simulink model "Vehicle_Model_Controller_may25"  (R2020b)
settings: Solver=VariableStepAuto  StartTime=0.0  StopTime=20  FixedStep=0.015  MaxStep=0.1  RelTol=1e-3
model workspace (MAT data in the model file):
  Kp = 10
  understeer_gradient = 0.05
undefined symbols (not defined in the file or in its folder): inch2mm, S1, S2, S3, S4, steer_slope
libraries: fl_lib x24, nesl_utility x22, sdl_lib x6, autolibshared x1, autolibdatasheetbattery x1, dspstat3 x1, pid_lib x1
(part 2 of 2)

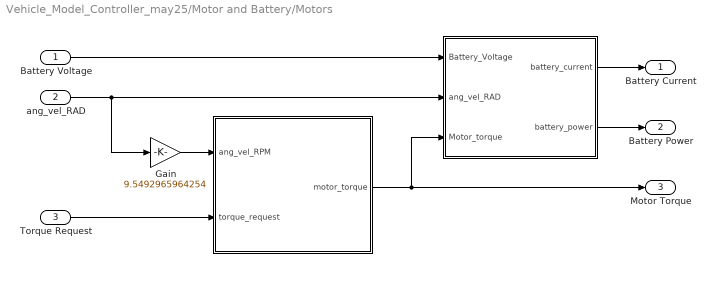
== system Vehicle_Model_Controller_may25/Motor and Battery/Motors ==
  Battery Voltage : Inport
  ang_vel_RAD : Inport  Port=2
  Torque Request : Inport  Port=3
  " " : MATLAB Function  TreatAsAtomicUnit=on
  "  " : MATLAB Function  TreatAsAtomicUnit=on
  Gain : Gain  Gain=9.5492965964254
  Battery Current : Outport
  Battery Power : Outport  Port=2
  Motor Torque : Outport  Port=3
  wires:
  Torque Request/1 -> " "/2(torque_request)
  Battery Voltage/1 -> "  "/1(Battery_Voltage)
  ang_vel_RAD/1 -> Gain/1, "  "/2(ang_vel_RAD)
  "  "/1(battery_current) -> Battery Current/1
  " "/1(motor_torque) -> Motor Torque/1, "  "/3(Motor_torque)
  "  "/2(battery_power) -> Battery Power/1
  Gain/1 -> " "/1(ang_vel_RPM)

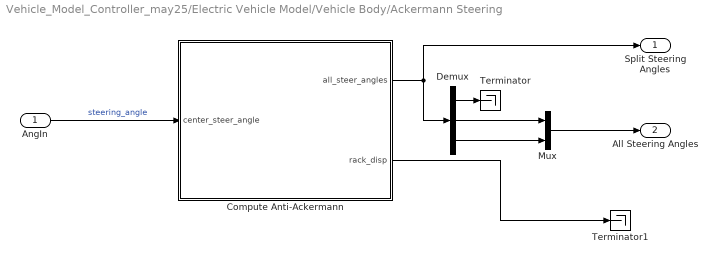
== system Vehicle_Model_Controller_may25/Electric Vehicle Model/Vehicle Body/Ackermann Steering ==
  AngIn : Inport
  Compute Anti-Ackermann : MATLAB Function  TreatAsAtomicUnit=on
  Demux : Demux  Outputs=3
  Mux : Mux  Inputs=2
  Terminator : Terminator
  Terminator1 : Terminator
  Split Steering Angles : Outport
  All Steering Angles : Outport  Port=2
  wires:
  Demux/1 -> Terminator/1
  Compute Anti-Ackermann/1(all_steer_angles) -> Demux/1, Split Steering Angles/1
  Demux/3 -> Mux/2
  AngIn/1 -> Compute Anti-Ackermann/1(center_steer_angle)  "steering_angle"
  Demux/2 -> Mux/1
  Mux/1 -> All Steering Angles/1
  Compute Anti-Ackermann/2(rack_disp) -> Terminator1/1

== matlab function Vehicle_Model_Controller_may25/Subsystem/MATLAB Function4 ==
  data: steering_angle input; torque_output output; torque_input_1 input size=[1 2]; torque_input_2 input size=[1 2]
function torque_output = cornering_torque_switcher(steering_angle, torque_input_1, torque_input_2)

if steering_angle ~= 0
    torque_output = torque_input_1;
else
    torque_output = torque_input_2;


end

== matlab function Vehicle_Model_Controller_may25/Subsystem/MATLAB Function3 ==
  data: vehicle_x_speed input; v output; vehicle_y_speed input
function v = fcn(vehicle_x_speed, vehicle_y_speed)

v = sqrt(vehicle_x_speed^2 + vehicle_y_speed^2);

== matlab function Vehicle_Model_Controller_may25/Electric Vehicle Model/Vehicle Body/Ackermann Steering/Compute Anti-Ackermann ==
  data: center_steer_angle input; all_steer_angles output size=[1 3]; S1 parameter; S2 parameter; S3 parameter; S4 parameter; inch2mm parameter; steer_slope parameter; deg2rad parameter; rack_disp output
function [all_steer_angles, rack_disp]  = anti_ackermann(center_steer_angle, S1, S2, S3, S4, inch2mm, steer_slope, deg2rad)
rack_disp = steer_slope * inch2mm * center_steer_angle;

left_steer_angle = -((S1*(-center_steer_angle)^3)+(S2*(-center_steer_angle)^2)+(S3*-center_steer_angle)+S4);
right_steer_angle = ((S1*(center_steer_angle)^3)+(S2*(center_steer_angle)^2)+(S3*center_steer_angle)+S4);

all_steer_angles = [center_steer_angle left_steer_angle right_steer_angle].*deg2rad;

end

== matlab function Vehicle_Model_Controller_may25/Motor and Battery/Motors/  ==
  data: ang_vel_RPM input; motor_torque output size=[1 2]; torque_request input
function motor_torque = get_torque(ang_vel_RPM, torque_request)
%% Actual Torque Output
% Developers:    Demetrius Gulewicz

% Developed for: Purdue Electric Racing
% Date:          09/18/2021
%
% Definitions:
% ang_vel:   Angular velocity of each wheel on the wheel fixed y axis [RPM]
% torque_request: Requested torque from the LP model                  [Nm]

%% Constants
% quadratic constants that connect current and max RPM of motors
a_v = 0.2667;
b_v = -66.353;
c_v = 10452 - ang_vel_RPM;

% quadratic constants that connnect current and max torque of motors
a_t = -0.0987;
b_t = 45.799;
c_t = -129.65;

% maximum possible current at the current RPM
max_current = [0, 0];


%% Calculate Maximum Torque Possible
% calculate the maximum current possible at the current RPM
for i = [1:2]
   if ang_vel_RPM(i) < 7000
       max_current(i) = 70;
   else
       max_current(i) = (-b_v - sqrt(b_v^2 - (4*a_v.*c_v(i)))) .* (1/(2*a_v));
   end
end

% calculate the meximum torque at the max current
max_torque = (a_t .* (max_current.^2)) + (b_t .* max_current) + c_t;
for i = [1:2]
   if max_torque(i) < 0
      max_torque(i) = 0;
   end
end

motor_torque_matrix = [max_torque; torque_request'];
motor_torque = min(motor_torque_matrix);

== matlab function Vehicle_Model_Controller_may25/Electric Vehicle Model/Vehicle Body/MATLAB Function ==
  data: Vy input; Vx input; Fext output
function Fext = get_downforce(Vy, Vx)
%% Constants
rho = 1.225; % Air density [Kg/m^3]
cl = 2.11014; % Lift coefficient [unitless]
A = 1.0221; % Frontal Area [m^2]


%% Computation
% Compute CoG Velocity
Vcog = Vx^2 + Vy^2;

% Compute DownForce
Fz = 0.5 * rho * Vcog * cl * A;
Fext = [0, 0, Fz];

== matlab function Vehicle_Model_Controller_may25/Electric Vehicle Model/MATLAB Function ==
  data: FwF output; FX input; FwR output
function [FwF, FwR] = fcn(FX)
%% Construct Force Matrix
FwF = FX(1:2);
FwR = FX(3:4);

== matlab function Vehicle_Model_Controller_may25/Subsystem/MATLAB Function ==
  data: driver_steering_angle output; vehicle_speed input; driver_steering_angle input; desired_wheelspeed output double
function [driver_steering_angle, desired_wheelspeed]  = wheel_speed_calculation(vehicle_speed, driver_steering_angle)
% desired_wheelspeed: 1 * 2 array [rl, rr]
% driver_steering_angle: 1 * angle variable
% vehicle_speed: 1 * VB CoG X-Velocity variable

W = 1.269; % m
L = 1.574; % m

ground_speed_rl = vehicle_speed + vehicle_speed * W * tan(driver_steering_angle) / (2*L);
ground_speed_rr = vehicle_speed - vehicle_speed * W * tan(driver_steering_angle) / (2*L);
desired_wheelspeed = [ground_speed_rl, ground_speed_rr];

== matlab function Vehicle_Model_Controller_may25/Subsystem/MATLAB Function1 ==
  data: measured_wheel_speed input; wheel_ground_speed output
function wheel_ground_speed = wheel_ground_speed_calculator(measured_wheel_speed)

% measured_wheel_speed: 1 * 4 array
% ackerman_angle      : 1 * 2 array

ground_speed_rl = measured_wheel_speed(5);
ground_speed_rr = measured_wheel_speed(6);

wheel_ground_speed = [ground_speed_rl, ground_speed_rr];

== matlab function Vehicle_Model_Controller_may25/Subsystem/MATLAB Function2 ==
  data: vel input; omega_m output size=[1 2]
function omega_m = wheel_angular_speed_calc(vel)
% motor shaft speed calculation, copied from Driver Input Logic/TV
% Controller/Layer_2

% a_theta: 1 * 2 ackermann steering angle
% vel:     1 * 6 measured wheel speed

r = 0.22; % Tire radius [m]
GR_r = (40/21) * (84/23) + 1; % Rear gear ratio [Unitless]
gr = [GR_r, GR_r]; % Gear ratios [Unitless]

% Motor Shaft Speed, RAD/S
omega_rl = vel(5);
omega_rr = vel(6);

omega_m = [omega_rl, omega_rr] .* (gr ./ r);

== matlab function Vehicle_Model_Controller_may25/Motor and Battery/Motors/   ==
  data: Battery_Voltage input; ang_vel_RAD input; battery_current output; Motor_torque input; battery_power output
function [battery_current, battery_power]= get_batt_curr(Battery_Voltage, ang_vel_RAD, Motor_torque)
%% Current Draw
% Developers:    Demetrius Gulewicz

% Developed for: Purdue Electric Racing
% Date:          09/18/2021
%
% Definitions:
% ang_vel_RAD:   Angular velocity of each wheel on the wheel fixed y axis [RAD]
% Motor_torque:  Torque the motor actually outputs                 [Ncm]
% Battery_Voltage: The voltage of the battery                      [V]

%% Definitions
a = 0.0411;
b = 2.7976;
c = 45.978;

t = Motor_torque;
w = ang_vel_RAD;
v = Battery_Voltage;

e = 85;

%% Calculate Current Draw
%x0 = [20, 20, 20, 20];
%options = optimoptions('fsolve','Algorithm','Levenberg-Marquardt');
%F = @(x) ([(a * x(1)^3) + (b * x(1)^2) + (c * x(1)), ] .* v) - (t .* w);
%battery_current = sum(fsolve(F,x0,options));

battery_current = sum((t .* w) ./ (e .* v));
battery_power = battery_current * Battery_Voltage;
end
